simulink model "affine_double_integrator"  (R2020b)
settings: Solver=ode4  StartTime=0.0  StopTime=50  FixedStep=0.01  RelTol=1e-3
InitFcn:
  | Initial_Parameters;
values from neighbouring files (symbols this model uses):
  kbeta = 1.5    [run_by_script.m]
  kp = 1    [run_by_script.m]
  kv = 10    [run_by_script.m]
  stressMat = -stressMat    [fcn_StressMatrix.m]
undefined symbols (not defined in the file or in its folder): acc_x, acc_y, c_y, delay, P0, w_y
settings Model: Creator=Fitz  LastModifiedBy=Fitz
settings DebuggingCC: UnderSpecifiedDimensionMsg=warning

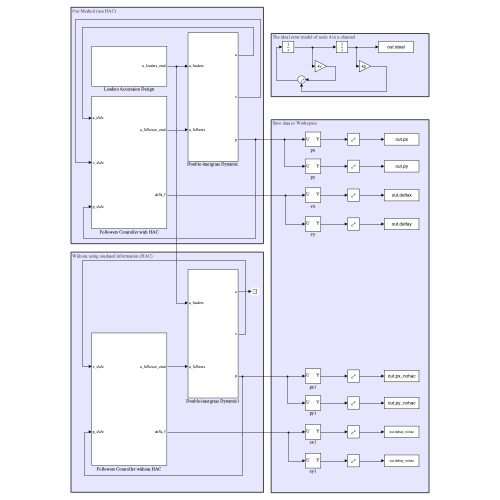
[thumbnail: Simulink's stored preview of the top-level diagram]
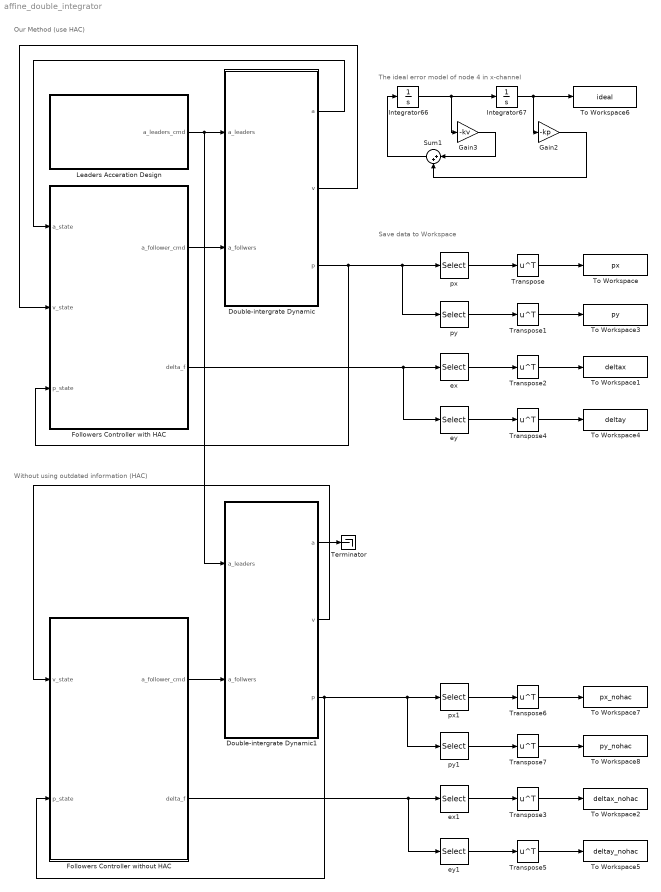
== system affine_double_integrator ==
  note: Save data to Workspace
  note: Our Method (use HAC)
  note: The ideal error model of node 4 in x-channel
  note: Without using outdated information (HAC)
  Double-intergrate Dynamic : Subsystem
  Double-intergrate Dynamic1 : Subsystem
  Followers Controller with HAC : Subsystem
  Followers Controller without HAC : Subsystem
  Gain2 : Gain  Gain=-kp
  Gain3 : Gain  Gain=-kv
  Integrator66 : Integrator
  Integrator67 : Integrator  InitialCondition=1
  Leaders Acceration Design : Subsystem
  Sum1 : Sum  Inputs=|++
  Terminator : Terminator
  To Workspace : ToWorkspace  VariableName=px  SampleTime=-1
      settings: Save2DSignal=2-D array (concatenate along first dimension)
  To Workspace1 : ToWorkspace  VariableName=deltax  SampleTime=-1
      settings: Save2DSignal=2-D array (concatenate along first dimension)
  To Workspace2 : ToWorkspace  VariableName=deltax_nohac  SampleTime=-1
      settings: Save2DSignal=2-D array (concatenate along first dimension)
  To Workspace3 : ToWorkspace  VariableName=py  SampleTime=-1
      settings: Save2DSignal=2-D array (concatenate along first dimension)
  To Workspace4 : ToWorkspace  VariableName=deltay  SampleTime=-1
      settings: Save2DSignal=2-D array (concatenate along first dimension)
  To Workspace5 : ToWorkspace  VariableName=deltay_nohac  SampleTime=-1
      settings: Save2DSignal=2-D array (concatenate along first dimension)
  To Workspace6 : ToWorkspace  VariableName=ideal  SampleTime=-1
      settings: Save2DSignal=2-D array (concatenate along first dimension)
  To Workspace7 : ToWorkspace  VariableName=px_nohac  SampleTime=-1
      settings: Save2DSignal=2-D array (concatenate along first dimension)
  To Workspace8 : ToWorkspace  VariableName=py_nohac  SampleTime=-1
      settings: Save2DSignal=2-D array (concatenate along first dimension)
  Transpose{,1..7} (8 alike) : Math  Operator=transpose  SaturateOnIntegerOverflow=on
  ex : Selector  NumberOfDimensions=2  InputPortWidth=3  IndexOptions=Select all,Index vector (dialog)  Indices=[1 3],1  OutputSizes=1,1
  ex1 : Selector  NumberOfDimensions=2  InputPortWidth=3  IndexOptions=Select all,Index vector (dialog)  Indices=[1 3],1  OutputSizes=1,1
  ey : Selector  NumberOfDimensions=2  InputPortWidth=3  IndexOptions=Select all,Index vector (dialog)  Indices=[1 3],2  OutputSizes=1,1
  ey1 : Selector  NumberOfDimensions=2  InputPortWidth=3  IndexOptions=Select all,Index vector (dialog)  Indices=[1 3],2  OutputSizes=1,1
  px : Selector  NumberOfDimensions=2  InputPortWidth=3  IndexOptions=Select all,Index vector (dialog)  Indices=[1 3],1  OutputSizes=1,1
  px1 : Selector  NumberOfDimensions=2  InputPortWidth=3  IndexOptions=Select all,Index vector (dialog)  Indices=[1 3],1  OutputSizes=1,1
  py : Selector  NumberOfDimensions=2  InputPortWidth=3  IndexOptions=Select all,Index vector (dialog)  Indices=[1 3],2  OutputSizes=1,1
  py1 : Selector  NumberOfDimensions=2  InputPortWidth=3  IndexOptions=Select all,Index vector (dialog)  Indices=[1 3],2  OutputSizes=1,1
  wires:
  Followers Controller with HAC/1(a_follower_cmd) -> Double-intergrate Dynamic/2(a_follwers)
  Leaders Acceration Design/1(a_leaders_cmd) -> Double-intergrate Dynamic1/1(a_leaders), Double-intergrate Dynamic/1(a_leaders)
  Double-intergrate Dynamic/1(a) -> Followers Controller with HAC/1(a_state)
  Double-intergrate Dynamic/2(v) -> Followers Controller with HAC/2(v_state)
  Double-intergrate Dynamic/3(p) -> Followers Controller with HAC/3(p_state), py/1, px/1
  Followers Controller with HAC/2(delta_f) -> ex/1, ey/1
  ex/1 -> Transpose2/1
  py/1 -> Transpose1/1
  px/1 -> Transpose/1
  Transpose/1 -> To Workspace/1
  Transpose1/1 -> To Workspace3/1
  Transpose2/1 -> To Workspace1/1
  ey/1 -> Transpose4/1
  Transpose4/1 -> To Workspace4/1
  Gain2/1 -> Sum1/2
  Integrator67/1 -> To Workspace6/1, Gain2/1
  Gain3/1 -> Sum1/1
  Integrator66/1 -> Gain3/1, Integrator67/1
  Sum1/1 -> Integrator66/1
  Followers Controller without HAC/1(a_follower_cmd) -> Double-intergrate Dynamic1/2(a_follwers)
  Double-intergrate Dynamic1/1(a) -> Terminator/1
  Double-intergrate Dynamic1/2(v) -> Followers Controller without HAC/1(v_state)
  Transpose5/1 -> To Workspace5/1
  Transpose3/1 -> To Workspace2/1
  ey1/1 -> Transpose5/1
  Followers Controller without HAC/2(delta_f) -> ey1/1, ex1/1
  ex1/1 -> Transpose3/1
  Transpose7/1 -> To Workspace8/1
  px1/1 -> Transpose6/1
  Double-intergrate Dynamic1/3(p) -> py1/1, px1/1, Followers Controller without HAC/2(p_state)
  Transpose6/1 -> To Workspace7/1
  py1/1 -> Transpose7/1

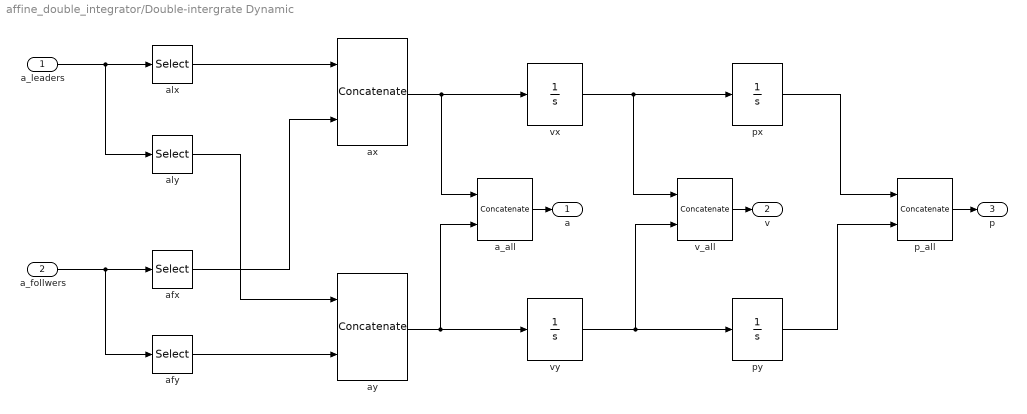
== system affine_double_integrator/Double-intergrate Dynamic ==
  a_leaders : Inport
  a_follwers : Inport  Port=2
  a_all : Concatenate  Mode=Multidimensional array  ConcatenateDimension=2
  afx : Selector  NumberOfDimensions=2  InputPortWidth=3  IndexOptions=Select all,Index vector (dialog)  Indices=[1 3],1  OutputSizes=1,1
  afy : Selector  NumberOfDimensions=2  InputPortWidth=3  IndexOptions=Select all,Index vector (dialog)  Indices=[1 3],2  OutputSizes=1,1
  alx : Selector  NumberOfDimensions=2  InputPortWidth=3  IndexOptions=Select all,Index vector (dialog)  Indices=[1 3],1  OutputSizes=1,1
  aly : Selector  NumberOfDimensions=2  InputPortWidth=3  IndexOptions=Select all,Index vector (dialog)  Indices=[1 3],2  OutputSizes=1,1
  ax : Concatenate  Mode=Multidimensional array
  ay : Concatenate  Mode=Multidimensional array
  p_all : Concatenate  Mode=Multidimensional array  ConcatenateDimension=2
  px : Integrator  InitialCondition=P0(:,1)
  py : Integrator  InitialCondition=P0(:,2)
  v_all : Concatenate  Mode=Multidimensional array  ConcatenateDimension=2
  vx : Integrator
  vy : Integrator
  a : Outport
  v : Outport  Port=2
  p : Outport  Port=3
  wires:
  a_leaders/1 -> aly/1, alx/1
  a_follwers/1 -> afx/1, afy/1
  alx/1 -> ax/1
  afx/1 -> ax/2
  afy/1 -> ay/2
  aly/1 -> ay/1
  ax/1 -> vx/1, a_all/1
  ay/1 -> vy/1, a_all/2
  a_all/1 -> a/1
  v_all/1 -> v/1
  vx/1 -> v_all/1, px/1
  vy/1 -> py/1, v_all/2
  px/1 -> p_all/1
  py/1 -> p_all/2
  p_all/1 -> p/1

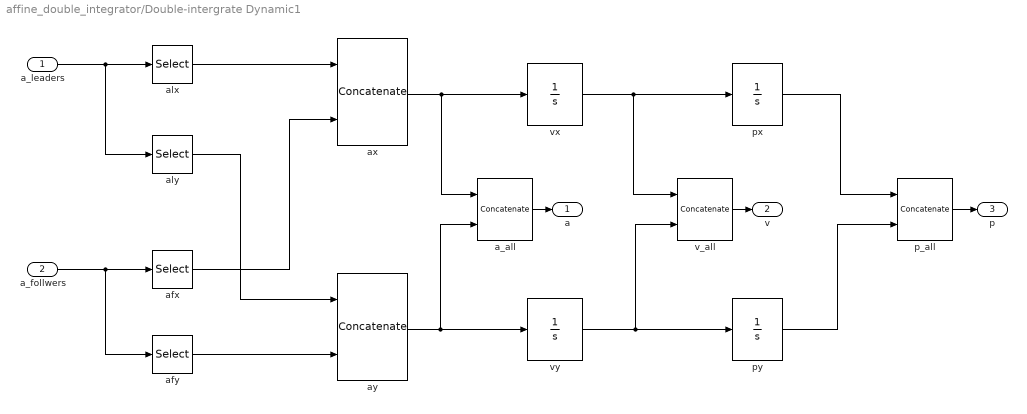
== system affine_double_integrator/Double-intergrate Dynamic1 ==
  a_leaders : Inport
  a_follwers : Inport  Port=2
  a_all : Concatenate  Mode=Multidimensional array  ConcatenateDimension=2
  afx : Selector  NumberOfDimensions=2  InputPortWidth=3  IndexOptions=Select all,Index vector (dialog)  Indices=[1 3],1  OutputSizes=1,1
  afy : Selector  NumberOfDimensions=2  InputPortWidth=3  IndexOptions=Select all,Index vector (dialog)  Indices=[1 3],2  OutputSizes=1,1
  alx : Selector  NumberOfDimensions=2  InputPortWidth=3  IndexOptions=Select all,Index vector (dialog)  Indices=[1 3],1  OutputSizes=1,1
  aly : Selector  NumberOfDimensions=2  InputPortWidth=3  IndexOptions=Select all,Index vector (dialog)  Indices=[1 3],2  OutputSizes=1,1
  ax : Concatenate  Mode=Multidimensional array
  ay : Concatenate  Mode=Multidimensional array
  p_all : Concatenate  Mode=Multidimensional array  ConcatenateDimension=2
  px : Integrator  InitialCondition=P0(:,1)
  py : Integrator  InitialCondition=P0(:,2)
  v_all : Concatenate  Mode=Multidimensional array  ConcatenateDimension=2
  vx : Integrator
  vy : Integrator
  a : Outport
  v : Outport  Port=2
  p : Outport  Port=3
  wires:
  a_leaders/1 -> aly/1, alx/1
  a_follwers/1 -> afx/1, afy/1
  alx/1 -> ax/1
  afx/1 -> ax/2
  afy/1 -> ay/2
  aly/1 -> ay/1
  ax/1 -> vx/1, a_all/1
  ay/1 -> vy/1, a_all/2
  a_all/1 -> a/1
  v_all/1 -> v/1
  vx/1 -> v_all/1, px/1
  vy/1 -> py/1, v_all/2
  px/1 -> p_all/1
  py/1 -> p_all/2
  p_all/1 -> p/1

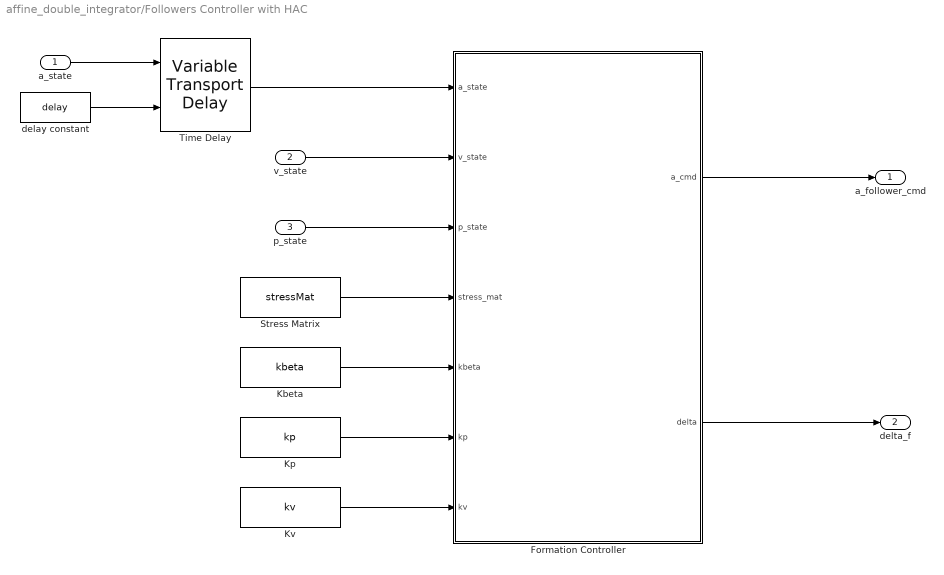
== system affine_double_integrator/Followers Controller with HAC ==
  a_state : Inport
  v_state : Inport  Port=2
  p_state : Inport  Port=3
  Formation Controller : MATLAB Function  TreatAsAtomicUnit=on
  Kbeta : Constant  Value=kbeta
  Kp : Constant  Value=kp
  Kv : Constant  Value=kv
  Stress Matrix : Constant  Value=stressMat
  Time Delay : VariableTransportDelay  MaximumDelay=10
  delay constant : Constant  Value=delay
  a_follower_cmd : Outport
  delta_f : Outport  Port=2
  wires:
  delay constant/1 -> Time Delay/2
  a_state/1 -> Time Delay/1
  Time Delay/1 -> Formation Controller/1(a_state)
  v_state/1 -> Formation Controller/2(v_state)
  p_state/1 -> Formation Controller/3(p_state)
  Stress Matrix/1 -> Formation Controller/4(stress_mat)
  Kbeta/1 -> Formation Controller/5(kbeta)
  Kp/1 -> Formation Controller/6(kp)
  Kv/1 -> Formation Controller/7(kv)
  Formation Controller/1(a_cmd) -> a_follower_cmd/1
  Formation Controller/2(delta) -> delta_f/1

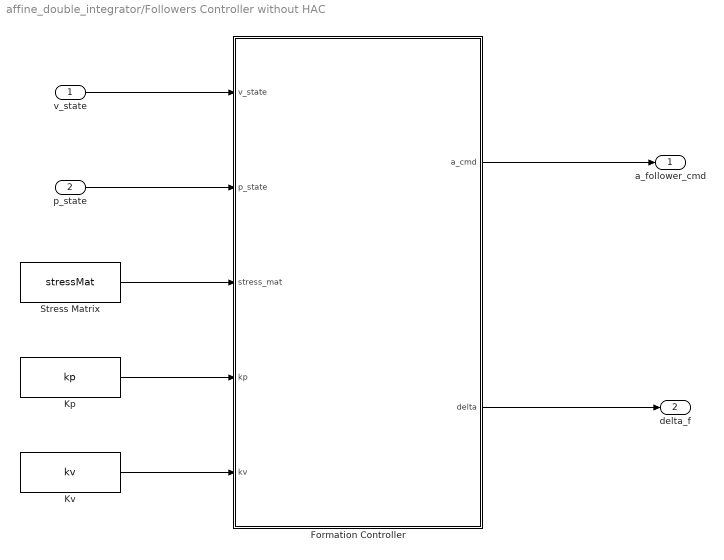
== system affine_double_integrator/Followers Controller without HAC ==
  v_state : Inport
  p_state : Inport  Port=2
  Formation Controller : MATLAB Function  TreatAsAtomicUnit=on
  Kp : Constant  Value=kp
  Kv : Constant  Value=kv
  Stress Matrix : Constant  Value=stressMat
  a_follower_cmd : Outport
  delta_f : Outport  Port=2
  wires:
  v_state/1 -> Formation Controller/1(v_state)
  p_state/1 -> Formation Controller/2(p_state)
  Stress Matrix/1 -> Formation Controller/3(stress_mat)
  Kp/1 -> Formation Controller/4(kp)
  Kv/1 -> Formation Controller/5(kv)
  Formation Controller/1(a_cmd) -> a_follower_cmd/1
  Formation Controller/2(delta) -> delta_f/1

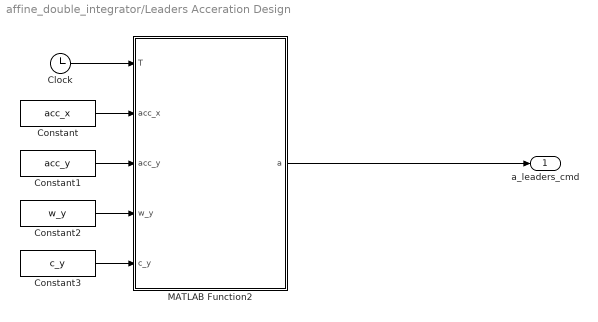
== system affine_double_integrator/Leaders Acceration Design ==
  Clock : Clock
  Constant : Constant  Value=acc_x
  Constant1 : Constant  Value=acc_y
  Constant2 : Constant  Value=w_y
  Constant3 : Constant  Value=c_y
  MATLAB Function2 : MATLAB Function  TreatAsAtomicUnit=on
  a_leaders_cmd : Outport
  wires:
  MATLAB Function2/1(a) -> a_leaders_cmd/1
  Clock/1 -> MATLAB Function2/1(T)
  Constant/1 -> MATLAB Function2/2(acc_x)
  Constant1/1 -> MATLAB Function2/3(acc_y)
  Constant2/1 -> MATLAB Function2/4(w_y)
  Constant3/1 -> MATLAB Function2/5(c_y)

== matlab function affine_double_integrator/Followers Controller without HAC/Formation Controller ==
  data: a_cmd output size=[followerNum, dim]; v_state input; p_state input; stress_mat input; kp input; kv input; delta output
function [a_cmd, delta] = formation_controller(v_state, p_state, stress_mat, kp, kv)
leaders_num = 3;
stressmat_ff = stress_mat(leaders_num+1:end,leaders_num+1:end);
stressmat_fl = stress_mat(leaders_num+1:end,1:leaders_num);
inv_stressmat_ff = inv(stressmat_ff);

delta = p_state(leaders_num+1:end,:) + inv_stressmat_ff * stressmat_fl * p_state(1:leaders_num,:);
E = stressmat_fl * p_state(1:leaders_num,:) + stressmat_ff * p_state(leaders_num+1:end,:);
dE = stressmat_fl * v_state(1:leaders_num,:) + stressmat_ff * v_state(leaders_num+1:end,:);

g = diag(stress_mat);
g(1:leaders_num) = [];

a_cmd = - (kp*E + kv*dE);
for i = 1:length(g)
    a_cmd(i,:) = a_cmd(i,:) / g(i);
end

== matlab function affine_double_integrator/Followers Controller with HAC/Formation Controller ==
  data: a_state input; a_cmd output size=[followerNum, dim]; v_state input; p_state input; stress_mat input; kbeta input; kp input; kv input; delta output
function [a_cmd, delta] = formation_controller(a_state, v_state, p_state, stress_mat, kbeta, kp, kv)
leaders_num = 3;
stressmat_ff = stress_mat(leaders_num+1:end,leaders_num+1:end);
stressmat_fl = stress_mat(leaders_num+1:end,1:leaders_num);
inv_stressmat_ff = inv(stressmat_ff);

delta = p_state(leaders_num+1:end,:) + inv_stressmat_ff * stressmat_fl * p_state(1:leaders_num,:);
E = stressmat_fl * p_state(1:leaders_num,:) + stressmat_ff * p_state(leaders_num+1:end,:);
dE = stressmat_fl * v_state(1:leaders_num,:) + stressmat_ff * v_state(leaders_num+1:end,:);
ddE = stressmat_fl * a_state(1:leaders_num,:) + stressmat_ff * a_state(leaders_num+1:end,:);

a_cmd = a_state(leaders_num+1:end,:) - kbeta * (kp*E + kv*dE + ddE);

== matlab function affine_double_integrator/Leaders Acceration Design/MATLAB Function2 ==
  data: T input; a output; acc_x input; acc_y input; w_y input; c_y input
function a = fcn_leaderV1(T,acc_x,acc_y,w_y,c_y)
leaders_num = 3;
a = zeros(leaders_num, 2);
current_time = T;

%% cos signal
ax = acc_x;
ay = acc_y*cos(w_y*current_time)+c_y;
% ay = a*sin(w*current_time)-a*cos(10*w*current_time)+c;

a(:,1) = ones(leaders_num, 1) * ax;
a(:,2) = ones(leaders_num, 1) * ay;
end
